simulink model "bpsk_rx6_PLL_based_Synchronization"  (R2020b)
settings: Solver=FixedStepDiscrete  StartTime=0.0  StopTime=2000  RelTol=1e-3
libraries: dsp_blocks x9
settings Model: Creator=hp  LastModifiedBy=hp

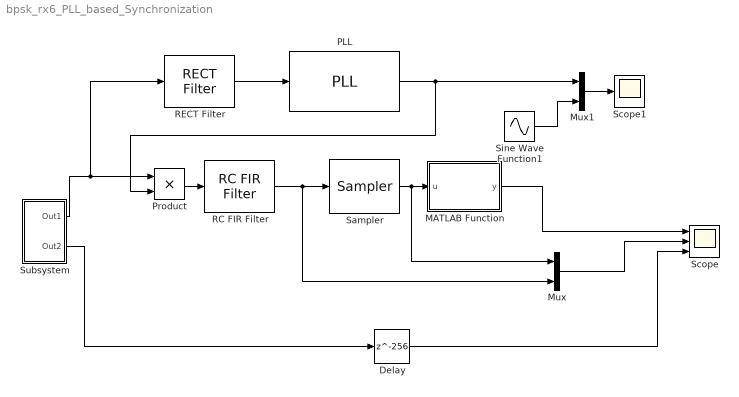
== system bpsk_rx6_PLL_based_Synchronization ==
  Delay : Delay  DelayLength=256
  MATLAB Function : MATLAB Function  TreatAsAtomicUnit=on
  Mux : Mux  Inputs=2
  Mux1 : Mux  Inputs=2
  PLL : dsp_blocks/Timing /PLL  freq=0.05  freq_out=0.1  phi=0  amp=2  xi=1  K=2  T=200
  Product : Product
  RC FIR Filter : dsp_blocks/Filters/RC FIR Filter  period=50  beta=0.5  root=on  filt_len=512  win_type=on
  RECT Filter : dsp_blocks/Filters/RECT Filter  f0=0.03  f1=0.07  filt_len=80
  Sampler : dsp_blocks/Conversions/Sampler  offset=512  samp_period=50
  Scope : Scope  NumInputPorts=3
  Scope1 : Scope
  Sine Wave Function1 : Sin  Amplitude=2  Frequency=2*pi*0.1  SampleTime=0
  Subsystem : Subsystem
  wires:
  Subsystem/1(Out1) -> RECT Filter/1, Product/1
  Subsystem/2(Out2) -> Delay/1
  Product/1 -> RC FIR Filter/1
  RC FIR Filter/1 -> Mux/2, Sampler/1
  Sampler/1 -> MATLAB Function/1(u), Mux/1
  MATLAB Function/1(y) -> Scope/1
  Mux/1 -> Scope/2
  Delay/1 -> Scope/3
  RECT Filter/1 -> PLL/1
  PLL/1 -> Product/2, Mux1/1
  Sine Wave Function1/1 -> Mux1/2
  Mux1/1 -> Scope1/1

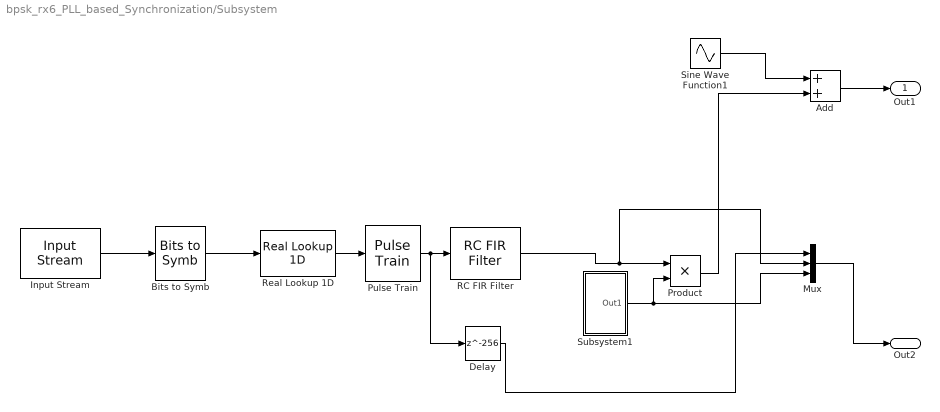
== system bpsk_rx6_PLL_based_Synchronization/Subsystem ==
  Add : Sum
  Bits to Symb : dsp_blocks/Conversions/Bits to Symb
  Delay : Delay  DelayLength=256
  Input Stream : dsp_blocks/Sources//Sinks/Input Stream  period=50  width=1  fname=rand.mat
  Mux : Mux  Inputs=3
  Product : Product
  Pulse Train : dsp_blocks/Conversions/Pulse Train  period=50
  RC FIR Filter : dsp_blocks/Filters/RC FIR Filter  period=50  beta=0.5  root=on  filt_len=512  win_type=on
  Real Lookup 1D : dsp_blocks/Conversions/Real Lookup 1D  table=[-1 1]
  Sine Wave Function1 : Sin  Amplitude=0.05  Frequency=2*pi*0.05  SampleTime=0
  Subsystem1 : Subsystem
  Out1 : Outport
  Out2 : Outport  Port=2
  wires:
  Real Lookup 1D/1 -> Pulse Train/1
  Pulse Train/1 -> Delay/1, RC FIR Filter/1
  RC FIR Filter/1 -> Mux/2, Product/1
  Subsystem1/1(Out1) -> Mux/3, Product/2
  Bits to Symb/1 -> Real Lookup 1D/1
  Input Stream/1 -> Bits to Symb/1
  Delay/1 -> Mux/1
  Mux/1 -> Out2/1
  Product/1 -> Add/2
  Add/1 -> Out1/1
  Sine Wave Function1/1 -> Add/1

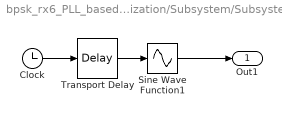
== system bpsk_rx6_PLL_based_Synchronization/Subsystem/Subsystem1 ==
  Clock : Clock
  Sine Wave Function1 : Sin  TimeSource=Use external signal  Amplitude=2  Frequency=2*pi*0.1  SampleTime=0
  Transport Delay : TransportDelay
  Out1 : Outport
  wires:
  Sine Wave Function1/1 -> Out1/1
  Transport Delay/1 -> Sine Wave Function1/1
  Clock/1 -> Transport Delay/1

== matlab function bpsk_rx6_PLL_based_Synchronization/MATLAB Function ==
  data: u input; y output
function y = fcn(u)
if (u > 0)
    y = 1;
else
    y = 0;
end
